simulink model "lab2statespace"  (R2014a)
settings: Solver=ode45  StartTime=0.0  StopTime=3.0  MaxStep=.001  RelTol=1e-3
values from neighbouring files (symbols this model uses):
  A = [-6 -25 ... (first row only)    [lab2code.m]
  B = [25 ... (first row only)    [lab2code.m]
  C = [1 0 ... (first row only)    [lab2code.m]
  D = [0 ... (first row only)    [lab2code.m]
settings Model: Creator=mmroman2  LastModifiedBy=mmroman2
settings DataIOCC: LimitDataPoints=off

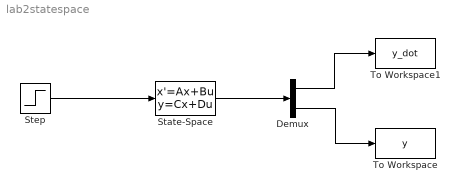
== system lab2statespace ==
  Demux : Demux  Outputs=2
  State-Space : StateSpace  A=A  B=B  C=C  D=D  X0=0
  Step : Step  Time=0  SampleTime=0
  To Workspace : ToWorkspace  VariableName=y  SampleTime=-1
  To Workspace1 : ToWorkspace  VariableName=y_dot  SampleTime=-1
  wires:
  State-Space/1 -> Demux/1
  Demux/1 -> To Workspace1/1
  Demux/2 -> To Workspace/1
  Step/1 -> State-Space/1
